simulink model "sim_all"  (R2020a)
settings: Solver=VariableStepAuto  StartTime=0.0  StopTime=2000  RelTol=1e-3
undefined symbols (not defined in the file or in its folder): a1, a2, alpha1, alpha2, cornerA, cornerB, cornerC, cornerD, ctrl_clockwise, ctrl_int_bound_or, ctrl_int_bound_pos, ctrl_k_or, ctrl_k_pos, ctrl_Ki_vel, ctrl_Kp_v_pos, ctrl_Kp_vel, ctrl_TAM, ctrl_Ts, ctrl_va_uncontrolled, ctrl_vel_uncontrolled, D, dead_zone_limit, depth, DiscIntNeverNeededParam, distanceFromWall, initInspectedSide, initPoint, mod_A, mod_Cd_F, mod_Cd_M, mod_eta_init, mod_g, mod_h0, mod_Ixx, mod_Iyy, mod_Izz, mod_Kp_dot, mod_lat0, mod_lon0, mod_m, mod_Mq_dot, mod_ni_init, mod_Nr_dot, mod_p1, mod_p2, mod_p3, mod_p4, mod_p5, mod_p6, mod_R, mod_Rm, mod_t1, mod_t2, mod_t3, mod_t4, mod_t5, mod_t6, mod_W, mod_Xu_dot, mod_Yv_dot ... (+53)
libraries: simulink x8, cstblocks x6, simulink_extras x1
(part 3 of 6)

== system sim_all/Mission_supervisor_v3/Mission_Supervisor/Orientazione Iniziale ==
  Pos_s : Inport
  Or_s : Inport  Port=2
  Or_in : Inport  Port=3
  error_flag : Inport  Port=4
  Action Port : ActionPort  ActionPortLabel=case [ 101 ]:
  Constant{,1..3} (4 alike) : Constant  Value=nan
  MATLAB Function : MATLAB Function  TreatAsAtomicUnit=on  SystemSampleTime=Ts_supervisor
  Mux : Mux  Inputs=6
  delta_current_or_iniz : Outport
  delta_stato_or_iniz : Outport  Port=2
  Outport : Outport  Port=3
  wires:
  MATLAB Function/2(delta_current_or_iniz) -> delta_current_or_iniz/1
  MATLAB Function/1(delta_stato_or_iniz) -> delta_stato_or_iniz/1
  Mux/1 -> Outport/1
  Constant/1 -> Mux/3
  Constant1/1 -> Mux/4
  Constant2/1 -> Mux/5
  Constant3/1 -> Mux/6
  Pos_s/1 -> MATLAB Function/1(Pos_s)
  Or_s/1 -> MATLAB Function/2(Or_s)
  Or_in/1 -> MATLAB Function/3(Or_in)
  MATLAB Function/3(Pos_d) -> Mux/1
  MATLAB Function/4(Or_d) -> Mux/2
  error_flag/1 -> MATLAB Function/4(error_flag)

== system sim_all/Mission_supervisor_v3/Mission_Supervisor/Orientazione in profondità ==
  Pos_s : Inport
  Orp_s : Inport  Port=2
  Punto_iniz_patt : Inport  Port=3
  error_flag : Inport  Port=4
  Action Port : ActionPort  ActionPortLabel=case [ 104 ]:
  Constant{,1..3,6} (5 alike) : Constant  Value=nan
  MATLAB Function : MATLAB Function  TreatAsAtomicUnit=on  SystemSampleTime=Ts_supervisor
  Mux : Mux  Inputs=6
  Mux1 : Mux  Inputs=3
  delta_current_or_prof : Outport
  delta_stato_or_prof : Outport  Port=2
  Outport : Outport  Port=3
  wires:
  MATLAB Function/1(delta_current_or_prof) -> delta_current_or_prof/1
  MATLAB Function/2(delta_stato_or_prof) -> delta_stato_or_prof/1
  MATLAB Function/3(Pos_d) -> Mux/1
  Mux/1 -> Outport/1
  Constant1/1 -> Mux/3
  MATLAB Function/4(Dpp_d) -> Mux/4
  MATLAB Function/5(Orp_d) -> Mux/6
  Constant/1 -> Mux1/1
  Constant2/1 -> Mux1/2
  Constant6/1 -> Mux1/3
  Mux1/1 -> Mux/2
  Constant3/1 -> Mux/5
  Pos_s/1 -> MATLAB Function/1(Pos_s)
  Orp_s/1 -> MATLAB Function/2(Orp_s)
  Punto_iniz_patt/1 -> MATLAB Function/3(punto_iniz_patt)
  error_flag/1 -> MATLAB Function/4(error_flag)

== system sim_all/Mission_supervisor_v3/Mission_Supervisor/Orientazione in superficie ==
  Or_in : Inport
  error_flag : Inport  Port=2
  punto_iniz_patt : Inport  Port=3
  Pos_s : Inport  Port=4
  Or_s : Inport  Port=5
  Action Port : ActionPort  ActionPortLabel=case [ 302 ]:
  Constant{1..2,4..5} (4 alike) : Constant  Value=nan
  MATLAB Function : MATLAB Function  TreatAsAtomicUnit=on  SystemSampleTime=Ts_supervisor
  Mux : Mux  Inputs=6
  delta_current_or_sup : Outport
  delta_stato_or_sup : Outport  Port=2
  Outport : Outport  Port=3
  wires:
  Mux/1 -> Outport/1
  Constant1/1 -> Mux/3
  Constant4/1 -> Mux/5
  Or_in/1 -> MATLAB Function/1(Or_in)
  error_flag/1 -> MATLAB Function/2(error_flag)
  punto_iniz_patt/1 -> MATLAB Function/3(punto_iniz_patt)
  MATLAB Function/1(delta_current_or_sup) -> delta_current_or_sup/1
  MATLAB Function/2(delta_stato_or_sup) -> delta_stato_or_sup/1
  MATLAB Function/4(Or_d) -> Mux/2
  MATLAB Function/3(Pos_d) -> Mux/1
  Constant2/1 -> Mux/4
  Constant5/1 -> Mux/6
  Pos_s/1 -> MATLAB Function/4(Pos_s)
  Or_s/1 -> MATLAB Function/5(Or_s)

== system sim_all/Mission_supervisor_v3/Mission_Supervisor/Pattugliamento ==
  parete : Inport
  contatore : Inport  Port=2
  Pos_s : Inport  Port=3
  Dpp_s : Inport  Port=4
  Dps_s : Inport  Port=5
  Orp_s : Inport  Port=6
  Vel_s : Inport  Port=7
  error_flag : Inport  Port=8
  giro : Inport  Port=9
  Action Port : ActionPort  ActionPortLabel=case [ 201 ]:
  Constant{,1..2,6} (4 alike) : Constant  Value=nan
  MATLAB Function : MATLAB Function  TreatAsAtomicUnit=on  SystemSampleTime=Ts_supervisor
  Mux : Mux  Inputs=6
  Mux1 : Mux  Inputs=3
  delta_current_patt : Outport
  delta_stato_patt : Outport  Port=2
  Outport : Outport  Port=3
  wires:
  MATLAB Function/1(delta_current_patt) -> delta_current_patt/1
  MATLAB Function/2(delta_stato_patt) -> delta_stato_patt/1
  parete/1 -> MATLAB Function/1(parete)
  contatore/1 -> MATLAB Function/2(contatore)
  MATLAB Function/3(Pos_d) -> Mux/1
  Mux/1 -> Outport/1
  Mux1/1 -> Mux/2
  MATLAB Function/4(Vel_d) -> Mux/3
  MATLAB Function/5(Dpp_d) -> Mux/4
  Constant/1 -> Mux1/1
  Constant2/1 -> Mux1/2
  Constant6/1 -> Mux1/3
  Pos_s/1 -> MATLAB Function/3(Pos_s)
  Dpp_s/1 -> MATLAB Function/4(Dpp_s)
  Dps_s/1 -> MATLAB Function/5(Dps_s)
  Vel_s/1 -> MATLAB Function/7(Vel_s)
  Orp_s/1 -> MATLAB Function/6(Orp_s)
  error_flag/1 -> MATLAB Function/8(error_flag)
  giro/1 -> MATLAB Function/9(giro)
  Constant1/1 -> Mux/5
  MATLAB Function/6(Orp_d) -> Mux/6

== system sim_all/Mission_supervisor_v3/Mission_Supervisor/Posizionamento ==
  Pos_s : Inport
  Or_s : Inport  Port=2
  punto iniziale : Inport  Port=3
  Or_in : Inport  Port=4
  error_flag : Inport  Port=5
  Action Port : ActionPort  ActionPortLabel=case [ 102 ]:
  Constant{,1..3} (4 alike) : Constant  Value=nan
  MATLAB Function : MATLAB Function  TreatAsAtomicUnit=on  SystemSampleTime=Ts_supervisor
  Mux : Mux  Inputs=6
  delta_current_posiz : Outport
  delta_stato_posiz : Outport  Port=2
  Outport : Outport  Port=3
  wires:
  MATLAB Function/1(delta_current_posiz) -> delta_current_posiz/1
  MATLAB Function/2(delta_stato_posiz) -> delta_stato_posiz/1
  MATLAB Function/3(Pos_d) -> Mux/1
  MATLAB Function/4(Or_d) -> Mux/2
  Mux/1 -> Outport/1
  Constant/1 -> Mux/3
  Constant1/1 -> Mux/6
  Constant2/1 -> Mux/5
  Pos_s/1 -> MATLAB Function/1(Pos_s)
  punto iniziale/1 -> MATLAB Function/3(punto_iniziale)
  Or_in/1 -> MATLAB Function/4(Or_in)
  Or_s/1 -> MATLAB Function/2(Or_s)
  error_flag/1 -> MATLAB Function/5(error_flag)
  Constant3/1 -> Mux/4

== system sim_all/Mission_supervisor_v3/Mission_Supervisor/Rientro ==
  Pos_s : Inport
  Or_in : Inport  Port=2
  error_flag : Inport  Port=3
  Dps_s : Inport  Port=4
  Dpp_s : Inport  Port=5
  Or_s : Inport  Port=6
  Action Port : ActionPort  ActionPortLabel=case [ 303 ]:
  Constant{1..4} (4 alike) : Constant  Value=nan
  MATLAB Function : MATLAB Function  TreatAsAtomicUnit=on  SystemSampleTime=Ts_supervisor
  Mux : Mux  Inputs=6
  delta_current_rient : Outport
  delta_stato_rient : Outport  Port=2
  Outport : Outport  Port=3
  wires:
  MATLAB Function/1(delta_current_rient) -> delta_current_rient/1
  MATLAB Function/2(delta_stato_rient) -> delta_stato_rient/1
  MATLAB Function/3(Pos_d) -> Mux/1
  Mux/1 -> Outport/1
  Constant1/1 -> Mux/3
  Constant2/1 -> Mux/4
  Constant3/1 -> Mux/5
  Constant4/1 -> Mux/6
  Pos_s/1 -> MATLAB Function/1(Pos_s)
  MATLAB Function/4(Or_d) -> Mux/2
  Or_in/1 -> MATLAB Function/2(Or_in)
  error_flag/1 -> MATLAB Function/3(error_flag)
  Dps_s/1 -> MATLAB Function/4(Dps_s)
  Dpp_s/1 -> MATLAB Function/5(Dpp_s)
  Or_s/1 -> MATLAB Function/6(Or_s)

== system sim_all/Mission_supervisor_v3/Mission_Supervisor/Risalita ==
  delta_SOS : Inport
  Pos_s : Inport  Port=2
  Dpp_s : Inport  Port=3
  Orp_s : Inport  Port=4
  Dps_s : Inport  Port=5
  Dps_fin : Inport  Port=6
  error_flag : Inport  Port=7
  SOS_205 : Inport  Port=8
  Action Port : ActionPort  ActionPortLabel=case [ 301 ]:
  Constant{,1,3,6} (4 alike) : Constant  Value=nan
  MATLAB Function : MATLAB Function  TreatAsAtomicUnit=on  SystemSampleTime=Ts_supervisor
  Mux : Mux  Inputs=6
  Mux1 : Mux  Inputs=3
  delta_current_ris : Outport
  delta_stato_ris : Outport  Port=2
  Outport : Outport  Port=3
  wires:
  MATLAB Function/1(delta_current_ris) -> delta_current_ris/1
  MATLAB Function/2(delta_stato_ris) -> delta_stato_ris/1
  MATLAB Function/3(Pos_d) -> Mux/1
  Mux/1 -> Outport/1
  Mux1/1 -> Mux/2
  Constant1/1 -> Mux/3
  MATLAB Function/4(Dpp_d) -> Mux/4
  Constant/1 -> Mux1/1
  Constant3/1 -> Mux1/2
  Constant6/1 -> Mux1/3
  MATLAB Function/5(Dps_d) -> Mux/5
  Pos_s/1 -> MATLAB Function/2(Pos_s)
  Dpp_s/1 -> MATLAB Function/3(Dpp_s)
  MATLAB Function/6(Orp_d) -> Mux/6
  delta_SOS/1 -> MATLAB Function/1(delta_SOS)
  Orp_s/1 -> MATLAB Function/4(Orp_s)
  Dps_s/1 -> MATLAB Function/5(Dps_s)
  Dps_fin/1 -> MATLAB Function/6(Dps_fin)
  error_flag/1 -> MATLAB Function/7(error_flag)
  SOS_205/1 -> MATLAB Function/8(SOS_205)

== system sim_all/Model/Vehicle Model/P1 ==
  note: n is the rotational speed of the thruster
      | V is the speed component of the water along the thruster axis
      |
      | n is saturated according to data
      | a dead zone is considered according to data
      | the thruster is characterised by 1st order dynamics (tau = 0.2s)
  n1 [rad/s] : Inport
  V1 [m/s] : Inport  Port=2
  Dead Zone : DeadZone  LowerValue=-dead_zone_limit  UpperValue=dead_zone_limit  SaturateOnIntegerOverflow=on
  Propeller1 : MATLAB Function  TreatAsAtomicUnit=on
  Saturation : Saturate  UpperLimit=n_max  LowerLimit=-n_max
  Transfer Fcn : TransferFcn  Denominator=[0.2 1]
  T1 : Outport
  wires:
  V1 [m/s]/1 -> Propeller1/2(V1)
  Saturation/1 -> Propeller1/1(n1)
  Transfer Fcn/1 -> Saturation/1
  Dead Zone/1 -> Transfer Fcn/1
  n1 [rad/s]/1 -> Dead Zone/1
  Propeller1/1(T1) -> T1/1

== system sim_all/Model/Vehicle Model/P2 ==
  note: n is the rotational speed of the thruster
      | V is the speed component of the water along the thruster axis
      |
      | n is saturated according to data
      | a dead zone is considered according to data
      | the thruster is characterised by 1st order dynamics (tau = 0.2s)
  n2 [rad/s] : Inport
  V2 [m/s] : Inport  Port=2
  Dead Zone : DeadZone  LowerValue=-dead_zone_limit  UpperValue=dead_zone_limit  SaturateOnIntegerOverflow=on
  Propeller2 : MATLAB Function  TreatAsAtomicUnit=on
  Saturation : Saturate  UpperLimit=n_max  LowerLimit=-n_max
  Transfer Fcn : TransferFcn  Denominator=[0.2 1]
  T2 : Outport
  wires:
  V2 [m/s]/1 -> Propeller2/2(V2)
  Saturation/1 -> Propeller2/1(n2)
  Transfer Fcn/1 -> Saturation/1
  Dead Zone/1 -> Transfer Fcn/1
  n2 [rad/s]/1 -> Dead Zone/1
  Propeller2/1(T2) -> T2/1

== system sim_all/Model/Vehicle Model/P3 ==
  note: n is the rotational speed of the thruster
      | V is the speed component of the water along the thruster axis
      |
      | n is saturated according to data
      | a dead zone is considered according to data
      | the thruster is characterised by 1st order dynamics (tau = 0.2s)
  n3 [rad/s] : Inport
  V3 [m/s] : Inport  Port=2
  Dead Zone : DeadZone  LowerValue=-dead_zone_limit  UpperValue=dead_zone_limit  SaturateOnIntegerOverflow=on
  Propeller3 : MATLAB Function  TreatAsAtomicUnit=on
  Saturation : Saturate  UpperLimit=n_max  LowerLimit=-n_max
  Transfer Fcn : TransferFcn  Denominator=[0.2 1]
  T3 : Outport
  wires:
  V3 [m/s]/1 -> Propeller3/2(V3)
  Saturation/1 -> Propeller3/1(n3)
  Transfer Fcn/1 -> Saturation/1
  Dead Zone/1 -> Transfer Fcn/1
  n3 [rad/s]/1 -> Dead Zone/1
  Propeller3/1(T3) -> T3/1

== system sim_all/Model/Vehicle Model/P4 ==
  note: n is the rotational speed of the thruster
      | V is the speed component of the water along the thruster axis
      |
      | n is saturated according to data
      | a dead zone is considered according to data
      | the thruster is characterised by 1st order dynamics (tau = 0.2s)
  n4 [rad/s] : Inport
  V4 [m/s] : Inport  Port=2
  Dead Zone : DeadZone  LowerValue=-dead_zone_limit  UpperValue=dead_zone_limit  SaturateOnIntegerOverflow=on
  Propeller4 : MATLAB Function  TreatAsAtomicUnit=on
  Saturation : Saturate  UpperLimit=n_max  LowerLimit=-n_max
  Transfer Fcn : TransferFcn  Denominator=[0.2 1]
  T4 : Outport
  wires:
  V4 [m/s]/1 -> Propeller4/2(V4)
  Saturation/1 -> Propeller4/1(n4)
  Transfer Fcn/1 -> Saturation/1
  Dead Zone/1 -> Transfer Fcn/1
  n4 [rad/s]/1 -> Dead Zone/1
  Propeller4/1(T4) -> T4/1

== system sim_all/Model/Vehicle Model/P5 ==
  note: n is the rotational speed of the thruster
      | V is the speed component of the water along the thruster axis
      |
      | n is saturated according to data
      | a dead zone is considered according to data
      | the thruster is characterised by 1st order dynamics (tau = 0.2s)
  n5 [rad/s] : Inport
  V5 [m/s] : Inport  Port=2
  Dead Zone : DeadZone  LowerValue=-dead_zone_limit  UpperValue=dead_zone_limit  SaturateOnIntegerOverflow=on
  Propeller5 : MATLAB Function  TreatAsAtomicUnit=on
  Saturation : Saturate  UpperLimit=n_max  LowerLimit=-n_max
  Transfer Fcn : TransferFcn  Denominator=[0.2 1]
  T5 : Outport
  wires:
  V5 [m/s]/1 -> Propeller5/2(V5)
  Saturation/1 -> Propeller5/1(n5)
  Transfer Fcn/1 -> Saturation/1
  Dead Zone/1 -> Transfer Fcn/1
  n5 [rad/s]/1 -> Dead Zone/1
  Propeller5/1(T5) -> T5/1

== system sim_all/Model/Vehicle Model/P6 ==
  note: n is the rotational speed of the thruster
      | V is the speed component of the water along the thruster axis
      |
      | n is saturated according to data
      | a dead zone is considered according to data
      | the thruster is characterised by 1st order dynamics (tau = 0.2s)
  n6 [rad/s] : Inport
  V6 [m/s] : Inport  Port=2
  Dead Zone : DeadZone  LowerValue=-dead_zone_limit  UpperValue=dead_zone_limit  SaturateOnIntegerOverflow=on
  Propeller6 : MATLAB Function  TreatAsAtomicUnit=on
  Saturation : Saturate  UpperLimit=n_max  LowerLimit=-n_max
  Transfer Fcn : TransferFcn  Denominator=[0.2 1]
  T6 : Outport
  wires:
  V6 [m/s]/1 -> Propeller6/2(V6)
  Saturation/1 -> Propeller6/1(n6)
  Transfer Fcn/1 -> Saturation/1
  Dead Zone/1 -> Transfer Fcn/1
  n6 [rad/s]/1 -> Dead Zone/1
  Propeller6/1(T6) -> T6/1

== system sim_all/Navigation/Extended Kalman Filter/AHRS__check ==
  AHRS_new : Inport
  MATLAB Function4 : MATLAB Function  TreatAsAtomicUnit=on
  Memory4 : Memory
  flag_AHRS : Outport
  AHRS_now : Outport  Port=2
  wires:
  AHRS_new/1 -> MATLAB Function4/1(AHRS_new)
  Memory4/1 -> MATLAB Function4/2(AHRS_old)
  MATLAB Function4/1(flag_AHRS) -> flag_AHRS/1
  MATLAB Function4/2(AHRS_now) -> Memory4/1, AHRS_now/1

== system sim_all/Navigation/Extended Kalman Filter/CORREZIONE ==
  x_k|k-1 : Inport
  P_k|k-1 : Inport  Port=2
  e : Inport  Port=3
  H : Inport  Port=4
  R : Inport  Port=5
  nav_flag_init : Inport  Port=6
  MATLAB Function : MATLAB Function  TreatAsAtomicUnit=on  SystemSampleTime=nav_DT
  x_k|k : Outport
  P_k|k : Outport  Port=2
  wires:
  x_k|k-1/1 -> MATLAB Function/1(x_k_k_1)
  P_k|k-1/1 -> MATLAB Function/2(P_k_k_1)
  e/1 -> MATLAB Function/3(e)
  H/1 -> MATLAB Function/4(H)
  MATLAB Function/1(x_k) -> x_k|k/1
  MATLAB Function/2(P_k) -> P_k|k/1
  nav_flag_init/1 -> MATLAB Function/6(nav_flag_init)
  R/1 -> MATLAB Function/5(R_k)

== system sim_all/Navigation/Extended Kalman Filter/DVL_check ==
  DVL_new : Inport
  MATLAB Function4 : MATLAB Function  TreatAsAtomicUnit=on
  Memory4 : Memory
  flag_DVL : Outport
  DVL_now : Outport  Port=2
  wires:
  DVL_new/1 -> MATLAB Function4/1(DVL_new)
  Memory4/1 -> MATLAB Function4/2(DVL_old)
  MATLAB Function4/1(flag_DVL) -> flag_DVL/1
  MATLAB Function4/2(DVL_now) -> Memory4/1, DVL_now/1

== system sim_all/Navigation/Extended Kalman Filter/MISURA VIRTUALE ==
  x_k|k-1 : Inport
  flag_vect : Inport  Port=2
  mis_vect : Inport  Port=3
  J : Inport  Port=4
  MATLAB Function : MATLAB Function  TreatAsAtomicUnit=on  SystemSampleTime=nav_DT
  e : Outport
  H : Outport  Port=2
  wires:
  x_k|k-1/1 -> MATLAB Function/1(x_k_k_1)
  mis_vect/1 -> MATLAB Function/3(mis_vect)
  flag_vect/1 -> MATLAB Function/2(flag_vect)
  MATLAB Function/1(e) -> e/1
  MATLAB Function/2(H) -> H/1
  J/1 -> MATLAB Function/4(J)

== system sim_all/Navigation/Extended Kalman Filter/PREDIZIONE ==
  x0 : Inport
  P0 : Inport  Port=2
  x_k-1|k-1 : Inport  Port=3
  u_k-1 : Inport  Port=4
  P_k-1|k-1 : Inport  Port=5
  J : Inport  Port=6
  L : Inport  Port=7
  Q_k-1 : Inport  Port=8
  nav_flag_init : Inport  Port=9
  Passo di Predizione : MATLAB Function  TreatAsAtomicUnit=on  SystemSampleTime=nav_DT
  x_k|k-1 : Outport
  P_k|k-1 : Outport  Port=2
  flag_init : Outport  Port=3
  wires:
  Passo di Predizione/1(x_k) -> x_k|k-1/1
  Passo di Predizione/2(P_k) -> P_k|k-1/1
  u_k-1/1 -> Passo di Predizione/4(u_k_1)
  x_k-1|k-1/1 -> Passo di Predizione/3(x_k_1)
  P_k-1|k-1/1 -> Passo di Predizione/5(P_k_1)
  J/1 -> Passo di Predizione/6(J)
  Q_k-1/1 -> Passo di Predizione/8(Q_k_1)
  P0/1 -> Passo di Predizione/2(P0)
  x0/1 -> Passo di Predizione/1(x0)
  L/1 -> Passo di Predizione/7(L)
  nav_flag_init/1 -> Passo di Predizione/9("nav_flag_init ")
  Passo di Predizione/3(nav_flag_init) -> flag_init/1

== system sim_all/Navigation/Extended Kalman Filter/Q_error ==
  flag_AHRS : Inport
  flag_DVL : Inport  Port=2
  Q : Inport  Port=3
  MATLAB Function4 : MATLAB Function  TreatAsAtomicUnit=on
  Memory : Memory
  Q_k : Outport
  wires:
  MATLAB Function4/1(Q_k) -> Q_k/1, Memory/1
  flag_AHRS/1 -> MATLAB Function4/3(flag_AHRS)
  flag_DVL/1 -> MATLAB Function4/4(flag_DVL)
  Memory/1 -> MATLAB Function4/2(Q_k_1)
  Q/1 -> MATLAB Function4/1(Q)

== system sim_all/Sensors/BLOCCO GYRO1/Subsystem ==
  t : Inport  SampleTime=sens_Sample_time_GYRO
  GEOD to NED : MATLAB Function  TreatAsAtomicUnit=on
  Bias_G : Outport
  wires:
  t/1 -> GEOD to NED/1(t)
  GEOD to NED/1(Bias_G) -> Bias_G/1

== matlab function sim_all/Navigation/Extended Kalman Filter/AHRS__check/MATLAB Function4 ==
  data: flag_AHRS output; AHRS_new input; AHRS_now output; AHRS_old input
%gestione di misura errata di AHRS
function [flag_AHRS, AHRS_now] = fcn(AHRS_new, AHRS_old)

    if isnan(AHRS_new(1,1)) || isnan(AHRS_new(2,1)) || isnan(AHRS_new(3,1))
        AHRS_now = AHRS_old;
        flag_AHRS = 1;
        disp('Misura AHRS non valida')
    else
        AHRS_now = AHRS_new;
        flag_AHRS = 0;
    end  
end

== matlab function sim_all/Navigation/Extended Kalman Filter/CORREZIONE/MATLAB Function ==
  data: x_k_k_1 input; x_k output; P_k_k_1 input; e input size=6 1; H input size=6 3; R_k input size=6 6; P_k output; nav_flag_init input
%%Passo di Correzione

function [x_k, P_k] = correction(x_k_k_1,P_k_k_1, e, H, R_k,nav_flag_init)
    
     x_k = zeros(3,1);
     P_k = zeros(3,3);
     
     
    if nav_flag_init ~= 0
        %matrice ottenuta da derivata di funzione h (6x1) per i rumori sei vari
        %sensori, che sono 6. (ha dimensione 6x6)
        %andrebbero anche considerati i rumori legati all'AHRS che al momento
        %sono trascurati
        %M = eye(6,6);              %M è l'dientità
        S_k = H*P_k_k_1*H'+ R_k;
        K_k = P_k_k_1*H'*(inv(S_k));

        P_k = (eye(3)-(K_k*H))*P_k_k_1;
        x_k = x_k_k_1 + K_k * e;
    end

end

== matlab function sim_all/Navigation/Extended Kalman Filter/Creazione vettore delle misure ==
  data: flag_vect output; GPS input; mis_vect output; depth input; s_pr input; s_dx input; s_sx input; mis_vect_prec input; J input; pos input; nav_plane_AB parameter; nav_plane_BC parameter; nav_plane_CD parameter; nav_plane_DA parameter; nav_A parameter; nav_B parameter; nav_C parameter; nav_D parameter; distanceFromWall parameter; flag_DVL input; flag_AHRS input
%%
% Questa funzione impila le informazioni derivanti dai vari sensori in un
% unico vettore mis_vect 7x1.                                 
% Ci sarà un corrispondente vettore flag_vect 7x1 di flag che sarà pari a:

% flag(i) = 0  se la misura è uguale a quella arrivata nell'istante
% predecente, in tal caso la correzione non verrà effettuata
% flag(i) = 1 se la misura è stata aggiornata rispetto a quella precendente
 
% NB il controllo sulla validità dei dati del GPS è valutata nel blocco
% sucessivo

function [flag_vect,mis_vect] = misure_vector(GPS,depth,s_pr,s_dx,s_sx, mis_vect_prec,...
          J, pos, nav_plane_AB, nav_plane_BC, nav_plane_CD, nav_plane_DA, nav_A, nav_B, nav_C, nav_D, distanceFromWall, ...
          flag_DVL, flag_AHRS)
    
    mis_vect = zeros(7,1);
    flag_vect = zeros(7,1);
	mis_vect = [GPS(1) GPS(2) GPS(3) depth s_pr s_dx s_sx]';
    
    for i=[1:7]
        if mis_vect(i) ~= mis_vect_prec(i)
            flag_vect(i) = 1;
        end
    end
    
    %si valuta se la misura del profondimetro è valida
    if isnan(depth)  
        flag_vect(4) = 0;
    end
     
    %si controlla che sia disponibile il dato dai sonar
    if isnan(s_pr)
        flag_vect(5) = 0;
    end
    if isnan(s_dx)
        flag_vect(6) = 0;
    end
    if isnan(s_sx)
        flag_vect(7) = 0;
    end
    
    %se i dati dei sonar qui sono utilizzabili, è necessario assicurarci che il 
    %loro raggio non punti verso uno spigolo, in quel caso potrebbe
    %causare una correzione errata
    if flag_vect(5) == 1               %se i dati del sonar di prua sono nuovi
            versore_son_NED = J*[1 0 0]';          %versore terna NED sonar prua
            flag_vect(5) = inter(pos, versore_son_NED ,nav_plane_AB,nav_plane_BC,nav_plane_CD,nav_plane_DA, nav_A, nav_B, nav_C, nav_D);       
    end

        if flag_vect(6) == 1               %se i dati del sonar destro sono nuovi
                versore_son_NED = J*[0 1 0]';          %versore terna NED sonar dx
                flag_vect(6) = inter(pos, versore_son_NED ,nav_plane_AB,nav_plane_BC,nav_plane_CD,nav_plane_DA, nav_A, nav_B, nav_C, nav_D);       
        end
        if flag_vect(7) == 1               %se i dati del sonar sinistro sono nuovi
                versore_son_NED = J*[0 -1 0]';          %versore terna NED sonar sx
                flag_vect(7) = inter(pos, versore_son_NED ,nav_plane_AB,nav_plane_BC,nav_plane_CD,nav_plane_DA, nav_A, nav_B, nav_C, nav_D);
        end 
%         la terza componente di flag_vect non sarà utilizzata. per assicurarci
%         che i dati del GPS siano validi ci rifaremo sempre su mis_vect


    if flag_DVL == 0 && flag_AHRS == 0  %i sonar vengono usati sempre nella correzione se un sensore tra DLV
                                        %o AHRS non funziona momentaneamente 
        
        soglia_distanza=distanceFromWall*3;
        soglia_variazione=0.8;
        if  mis_vect(5) > soglia_distanza || abs(mis_vect(5)- mis_vect_prec(5)) > soglia_variazione
            flag_vect(5) = 0;
        end
        if  mis_vect(6) > soglia_distanza || abs(mis_vect(6)- mis_vect_prec(6)) > soglia_variazione
            flag_vect(6) = 0;
        end
        if  mis_vect(7) > soglia_distanza || abs(mis_vect(7)- mis_vect_prec(7)) > soglia_variazione
            flag_vect(7) = 0;
        end
    end
end




function [flag] = inter(pos, versore_son_NED,nav_plane_AB,nav_plane_BC,nav_plane_CD,nav_plane_DA, nav_A, nav_B, nav_C, nav_D)
    
    %calcolo della distanza dalla posizione ai piani delle pareti seguendo
    %la direzione data dal versore del sonar

    t_AB = -(pos(1)+nav_plane_AB(2)*pos(2)+nav_plane_AB(4))/(nav_plane_AB(2)*versore_son_NED(2)+versore_son_NED(1));
    t_BC = -(pos(1)+nav_plane_BC(2)*pos(2)+nav_plane_BC(4))/(nav_plane_BC(2)*versore_son_NED(2)+versore_son_NED(1));
    t_CD = -(pos(1)+nav_plane_CD(2)*pos(2)+nav_plane_CD(4))/(nav_plane_CD(2)*versore_son_NED(2)+versore_son_NED(1));
    t_DA = -(pos(1)+nav_plane_DA(2)*pos(2)+nav_plane_DA(4))/(nav_plane_DA(2)*versore_son_NED(2)+versore_son_NED(1));
    
    if t_AB < 0
        t_AB = inf;
    end
    if t_BC < 0
        t_BC = inf;
    end
    if t_CD < 0
        t_CD = inf;
    end
    if t_DA < 0
        t_DA = inf;
    end
           
    [dist, index] = min([t_AB t_BC t_CD t_DA]);
    dist = dist - 0.267;       %va tolto il raggio del veicolo rispetto al centro di massa
    
    int=zeros(1,3);
    %calcolo l'intersezione
    int(1) = pos(1) + versore_son_NED(1)*dist;
    int(2) = pos(2) + versore_son_NED(2)*dist;
    int(3) = 0;
    
    soglia_spigolo = 5;          %distanza massima dallo spigolo entro la quale 
                       %la misura del sonar non è buona
    flag=1;
    switch index
        case 1      
            if norm(int-nav_A) < soglia_spigolo || norm(int-nav_B) < soglia_spigolo
                flag=0;
            end
        case 2
            if norm(int-nav_B) < soglia_spigolo || norm(int-nav_C) < soglia_spigolo
                flag=0;
            end
        case 3
            if norm(int-nav_C) < soglia_spigolo || norm(int-nav_D) < soglia_spigolo
                flag=0;
            end
        case 4
            if norm(int-nav_D) < soglia_spigolo || norm(int-nav_A) < soglia_spigolo
                flag=0;
            end
        otherwise
            disp('errore nella intersezione del piano')
    end
end

== matlab function sim_all/Mission_supervisor_v3/Mission_Supervisor/Orientazione Iniziale/MATLAB Function ==
  data: delta_stato_or_iniz output; delta_current_or_iniz output; Pos_d output size=3; Pos_s input size=3; Or_s input size=3; Or_in input; initPoint parameter size=3; Or_d output size=3; error_flag input; soglia_or parameter; soglia_SOS_pos parameter; SOS parameter; soglia_SOS_or parameter
function [delta_stato_or_iniz, delta_current_or_iniz, Pos_d, Or_d] = Orientazione_iniziale(Pos_s, Or_s, Or_in, initPoint, error_flag, soglia_or, soglia_SOS_pos, SOS, soglia_SOS_or)

    disp("Orientazione iniziale");
    
    %% Unità di misura 
    
    % Pos_d, Pos_s, initPoint, soglia_SOS_pos                                [deg, deg, m]
    % Or_d, Or_s, Or_in, soglia_or, soglia_SOS_or                            [rad, rad, rad]
    
    %% Inizializzazione variabili
    
    % Mantenimento dello stato_interno al valore
    % desiderato durante la permanenza del sistema nello stato corrente.
    delta_stato_or_iniz = 0;
    
    % Variabile utilizzata per segnalare il momento in cui
    % effettuare la transizione di stato. 
    pronti = false;
    
    %% Preparazione dei riferimenti da fornire ai blocchi successivi
                
    % Posizione da mantenere
    Pos_d = initPoint; 
   
    % Orientazione desiderata per raggiungere
    % il punto di inizio pattugliamento
    Or_d = Or_in;
    
    % Quando i riferimenti sono correttamente settati
    % il passaggio di stato viene comunicato agli altri moduli
    delta_current_or_iniz = 101 - 100;
    
    
    %% Verifiche
    
    % Si verifica il mantenimento della posizione 
    % e la ricezione della stima di orientazione
    if (abs(Pos_s(1) - Pos_d(1)) > soglia_SOS_pos(1) || ...
        abs(Pos_s(2) - Pos_d(2)) > soglia_SOS_pos(2) || ...
        abs(Pos_s(3) - Pos_d(3)) > soglia_SOS_pos(3) || ...
        isnan(Or_s(1)) || isnan(Or_s(2)) || isnan(Or_s(3)) || ...
        abs(Or_s(1) - Or_d(1)) > soglia_SOS_or(1) || ...
        abs(Or_s(2) - Or_d(2)) > soglia_SOS_or(2))
    
        SOS = 1;
        disp("EMERGENZA:");
        
        if (abs(Pos_s(1) - Pos_d(1)) > soglia_SOS_pos(1))
            disp("Rilevato errore sulla posizione X");
        end
        if (abs(Pos_s(2) - Pos_d(2)) > soglia_SOS_pos(2))
            disp("Rilevato errore sulla posizione Y");
        end
        if (abs(Pos_s(3) - Pos_d(3)) > soglia_SOS_pos(3))
            disp("Rilevato errore sulla profondita Z");
        end
        if (isnan(Or_s(1)))
            disp("Mancata ricezione della prima componente di orientazione");
        end
        if (isnan(Or_s(2)))
            disp("Mancata ricezione della seconda componente di orientazione");
        end
        if (isnan(Or_s(3)))
            disp("Mancata ricezione della terza componente di orientazione");
        end
        if (abs(Or_s(1) - Or_d(1)) > soglia_SOS_or(1))
            disp("Rilevato errore sulla rotazione di roll");
        end
        if (abs(Or_s(2) - Or_d(2)) > soglia_SOS_or(2))
            disp("Rilevato errore sulla rotazione di pitch");
        end
    end

    if error_flag == 1
        disp("EMERGENZA: errore segnalato dagli altri sottosistemi");
        SOS = 1;
    end
    
    % Si verifica di aver raggiunto l'orientazione desiderata
    if (SOS == 0 && ...
        (abs(Or_s(3) - Or_d(3)) < soglia_or(3)))
    
        pronti = true;
        
    end
       
    %% Decisione dello stato successivo
    
    if pronti == true
        
        delta_stato_or_iniz = 102 - 101; % Transizione eseguita correttamente
    end
        
    if SOS == 1
            
            delta_stato_or_iniz = 304 - 101; % Transizione nello stato di emergenza
    end
    % Si rimane nello stato corrente

end

== matlab function sim_all/Navigation/Extended Kalman Filter/DVL_check/MATLAB Function4 ==
  data: flag_DVL output; DVL_new input; DVL_now output; DVL_old input
%gestione di misura errata del DVL
function [flag_DVL, DVL_now] = fcn(DVL_new, DVL_old)

    if isnan(DVL_new(1,1)) || isnan(DVL_new(2,1)) || isnan(DVL_new(3,1))
        DVL_now = DVL_old;
        flag_DVL = 1;
        disp('Misura DVL non valida')
    else
        DVL_now = DVL_new;
        flag_DVL = 0;
    end  
end

== matlab function sim_all/Navigation/Extended Kalman Filter/MATLAB Function ==
  data: GPS input; x0 output; depth input; P0 output; flag input; flag output
%blocco di inizializzazione del Filtro

function [x0, P0, flag] = EKF_init(GPS, depth, flag)
    
    x0 = zeros(3,1);
    P0 = zeros(3,3);
    
    % il valore di nav_flag_init è all'inizio della simulazione pari a 0
    % appena c'è il primo dato disponibile del GPS (insieme al profondimetro)
    % si assume quella come punto di inizializzazione del filtro.

    if flag == 0
        if GPS(3)==1
            x0 = [GPS(1), GPS(2), depth]';
            P0 = diag([3 3 (0.2)^2]);       %sono le varianze del GPS e del profondimetro (come nella R)
            flag = 1;                   %se vale 1 bisogna assegnare i primi valori a x_k_1 e P_k_1
        end
               
    end

end

== matlab function sim_all/Navigation/Extended Kalman Filter/MATLAB Function1 ==
  data: orient input; J output
%calcolo matrice J
function J = calcolo_jacobiano(orient)

    Roll  = orient(1);
    Pitch = orient(2);
    Yaw   = orient(3);

    R_x = [ 1               0              0;
            0           cos(Roll)     sin(Roll);
            0           -sin(Roll)    cos(Roll)];

    R_y = [cos(Pitch)       0   -sin(Pitch);
              0             1         0;
           sin(Pitch)       0   cos(Pitch)];

    R_z = [cos(Yaw)     sin(Yaw)      0;
          -sin(Yaw)     cos(Yaw)      0;
              0            0          1];

    J = (R_z'*R_y')*R_x';
end

== matlab function sim_all/Navigation/Extended Kalman Filter/MATLAB Function2 ==
  data: u_k_1 input; orient input; L output
%calcolo matrice L
function L = calcolo_L(u_k_1,orient)

    L =  [   u_k_1(2)*((sin(orient(1))*sin(orient(3)))/10 + (cos(orient(1))*cos(orient(3))*sin(orient(2)))/10) + u_k_1(3)*((cos(orient(1))*sin(orient(3)))/10 - (cos(orient(3))*sin(orient(1))*sin(orient(2)))/10), (u_k_1(3)*cos(orient(1))*cos(orient(3))*cos(orient(2)))/10 - (u_k_1(1)*cos(orient(3))*sin(orient(2)))/10 + (u_k_1(2)*cos(orient(3))*cos(orient(2))*sin(orient(1)))/10, u_k_1(3)*((cos(orient(3))*sin(orient(1)))/10 - (cos(orient(1))*sin(orient(3))*sin(orient(2)))/10) - u_k_1(2)*((cos(orient(1))*cos(orient(3)))/10 + (sin(orient(1))*sin(orient(3))*sin(orient(2)))/10) - (u_k_1(1)*cos(orient(2))*sin(orient(3)))/10, (cos(orient(3))*cos(orient(2)))/10, (cos(orient(3))*sin(orient(1))*sin(orient(2)))/10 - (cos(orient(1))*sin(orient(3)))/10, (sin(orient(1))*sin(orient(3)))/10 + (cos(orient(1))*cos(orient(3))*sin(orient(2)))/10;...
           - u_k_1(2)*((cos(orient(3))*sin(orient(1)))/10 - (cos(orient(1))*sin(orient(3))*sin(orient(2)))/10) - u_k_1(3)*((cos(orient(1))*cos(orient(3)))/10 + (sin(orient(1))*sin(orient(3))*sin(orient(2)))/10), (u_k_1(3)*cos(orient(1))*cos(orient(2))*sin(orient(3)))/10 - (u_k_1(1)*sin(orient(3))*sin(orient(2)))/10 + (u_k_1(2)*cos(orient(2))*sin(orient(1))*sin(orient(3)))/10, u_k_1(3)*((sin(orient(1))*sin(orient(3)))/10 + (cos(orient(1))*cos(orient(3))*sin(orient(2)))/10) - u_k_1(2)*((cos(orient(1))*sin(orient(3)))/10 - (cos(orient(3))*sin(orient(1))*sin(orient(2)))/10) + (u_k_1(1)*cos(orient(3))*cos(orient(2)))/10, (cos(orient(2))*sin(orient(3)))/10, (cos(orient(1))*cos(orient(3)))/10 + (sin(orient(1))*sin(orient(3))*sin(orient(2)))/10, (cos(orient(1))*sin(orient(3))*sin(orient(2)))/10 - (cos(orient(3))*sin(orient(1)))/10;...
                                                                                                             (u_k_1(2)*cos(orient(1))*cos(orient(2)))/10 - (u_k_1(3)*cos(orient(2))*sin(orient(1)))/10,                                      - (u_k_1(1)*cos(orient(2)))/10 - (u_k_1(3)*cos(orient(1))*sin(orient(2)))/10 - (u_k_1(2)*sin(orient(1))*sin(orient(2)))/10,                                                                                                                                                                                                                              0,               -sin(orient(2))/10,                                               (cos(orient(2))*sin(orient(1)))/10,                                               (cos(orient(1))*cos(orient(2)))/10]; 
end

== matlab function sim_all/Navigation/Extended Kalman Filter/MATLAB Function3 ==
  data: flag_vect input; mis_vect input; R_ input size=6 6; R_k output size=6 6
%calcolo matrice R
function R_k = R_cutter(flag_vect, mis_vect,R_)
%valutazione misure GPS
    R=R_;   
    i=0;
    if mis_vect(3) == 0                    %se i dati del GPS non sono validi
        R(1,:) = [];
        R(:,1) = [];
        i=i+1;
        R(2-i,:) = [];
        R(:,2-i) = [];
        i=i+1;
        if flag_vect(4) == 0               %se i dati del profondimetro non sono nuovi
            R(3-i,:) = [];
            R(:,3-i) = [];
            i=i+1;
        end
        if flag_vect(5) == 0               %se i dati del sonar di prua non sono nuovi
            R(4-i,:) = [];
             R(:,4-i) = [];
            i=i+1;
        end
        if flag_vect(6) == 0               %se i dati del sonar sinistro non sono nuovi
            R(5-i,:) = [];
             R(:,5-i) = [];
            i=i+1;
        end
        if flag_vect(7) == 0               %se i dati del sonar destro non sono nuovi
            R(6-i,:) = [];
             R(:,6-i) = [];
        end
    % da qui invece abbiamo il GPS valido
    else
        if flag_vect(1)==0 || flag_vect(2)==0  %se i dati del GPS non sono nuovi
            R(1-i,:) = [];
            R(:,1-i) = [];
            i=i+1;
            R(2-i,:) = [];
            R(:,2-i) = [];
            i=i+1;
        end
       
        if flag_vect(4) == 0               %se i dati del profondimetro non sono nuovi
            R(3-i,:) = [];
            R(:,3-i) = [];
            i=i+1;
        end
       
        R(4-i,:) = []; %annulliamo le misure dei sonar
        R(:,4-i) = [];         
        i=i+1;
        R(5-i,:) = [];
        R(:,5-i) = [];
        i=i+1;
        R(6-i,:) = [];
        R(:,6-i) = [];
       
    end
    R_k=R;
end

== matlab function sim_all/Navigation/Extended Kalman Filter/MISURA VIRTUALE/MATLAB Function ==
  data: x_k_k_1 input; flag_vect input; mis_vect input; e output size=6 1; H output size=6 3; J input; nav_plane_AB parameter; nav_plane_BC parameter; nav_plane_CD parameter; nav_plane_DA parameter
%calcolo  misure virtuali
function [e, H] = virtual(x_k_k_1, flag_vect, mis_vect, J, nav_plane_AB, nav_plane_BC, nav_plane_CD, nav_plane_DA)

    e = zeros(6,1);
    h = zeros(6,1);
    z = zeros(6,1);
    H = zeros(6,3);
    
    
    %valutazione misure GPS
    if mis_vect(3)==1                                   %se i dati del GPS sono validi
        if flag_vect(1) == 1 && flag_vect(2) == 1       %se i dati del GPS sono nuovi
            
            z = z + [mis_vect(1) mis_vect(2) 0 0 0 0]';
            h = h + [x_k_k_1(1)   x_k_k_1(2) 0 0 0 0]';
        
            H(1,:)= [1 0 0];
            H(2,:)= [0 1 0];
        end
    end
    
    %valutazione misure depth
    if flag_vect(4) == 1                                 %se i dati del profondimetro sono nuovi
            
        z = z + [0 0 mis_vect(4) 0 0 0]'; 
        h = h + [0 0  x_k_k_1(3) 0 0 0]';

        H(3,:)= [0 0 1];
    end
    
    %valutiamo ora le misure virtuali solo se quelle del GPS non sono
    %valide
    if mis_vect(3)==0                      %se i dati del GPS non sono validi
        
        if flag_vect(5) == 1               %se i dati del sonar di prua sono nuovi
                
                versore_son_NED = J*[1 0 0]';          %versore terna NED sonar prua
                
                [distanza, plane] = inter(x_k_k_1, versore_son_NED ,nav_plane_AB,nav_plane_BC,nav_plane_CD,nav_plane_DA);
                z = z + [0 0 0 mis_vect(5) 0 0]'; 
                h = h + [0 0 0 distanza    0 0]';
                
                H_new=zeros(1,3);
                [H_new(1), H_new(2), H_new(3)] = calc_H_vect(x_k_k_1, versore_son_NED,plane);
                H(4,:) = H_new;                
        end
    
        if flag_vect(6) == 1               %se i dati del sonar destro sono nuovi
                
                versore_son_NED = J*[0 1 0]';          %versore terna NED sonar dx
                
                [distanza, plane] = inter(x_k_k_1, versore_son_NED ,nav_plane_AB,nav_plane_BC,nav_plane_CD,nav_plane_DA);
                z = z + [0 0 0 0 mis_vect(6) 0]'; 
                h = h + [0 0 0 0 distanza    0]';
                
                H_new=zeros(1,3);
                [H_new(1), H_new(2), H_new(3)] = calc_H_vect(x_k_k_1, versore_son_NED,plane);
                H(5,:) = H_new;
        end
    
        if flag_vect(7) == 1               %se i dati del sonar sinistro sono nuovi
                 
                versore_son_NED = J*[0 -1 0]';          %versore terna NED sonar sx
                
                [distanza, plane] = inter(x_k_k_1, versore_son_NED ,nav_plane_AB,nav_plane_BC,nav_plane_CD,nav_plane_DA);
                z = z + [0 0 0 0 0 mis_vect(7)]'; 
                h = h + [0 0 0 0 0 distanza   ]'; 
                
                H_new=zeros(1,3);
                [H_new(1), H_new(2), H_new(3)] = calc_H_vect(x_k_k_1, versore_son_NED,plane);
                H(6,:) = H_new;
        end
    end
    
    e = z - h;
    
    %%si riducono le dimensioni della matrice H e del vettore e
    
    i=0;
    if mis_vect(3) == 0                    %se i dati del GPS non sono validi
        H(1-i,:) = [];
        e(1-i) = [];
        i=i+1;
        H(2-i,:) = [];
        e(2-i) = [];
        i=i+1;
        if flag_vect(4) == 0               %se i dati del profondimetro non sono nuovi
            H(3-i,:) = [];
            e(3-i) = [];
            i=i+1;
        end
        if flag_vect(5) == 0               %se i dati del sonar di prua non sono nuovi
            H(4-i,:) = [];
            e(4-i) = [];
            i=i+1;
        end
        if flag_vect(6) == 0               %se i dati del sonar sinistro non sono nuovi
            H(5-i,:) = [];
            e(5-i) = [];
            i=i+1;
        end
        if flag_vect(7) == 0               %se i dati del sonar destro non sono nuovi
            H(6-i,:) = [];
            e(6-i) = [];
        end
    % da qui invece si ha il GPS valido
    else
        if flag_vect(1)==0 || flag_vect(2)==0  %se i dati del GPS non sono nuovi
            H(1-i,:) = [];
            e(1-i) = [];
            i=i+1;
            H(2-i,:) = [];
            e(2-i) = [];
            i=i+1;
        end
        
        if flag_vect(4) == 0               %se i dati del profondimetro non sono nuovi
            H(3-i,:) = [];
            e(3-i) = [];
            i=i+1;
        end
        
        H(4-i,:) = [];                      %annulliamo le misure dei sonar
        e(4-i) = [];
        i=i+1;
        H(5-i,:) = [];
        e(5-i) = [];
        i=i+1;
        H(6-i,:) = [];        
        e(6-i) = [];    
    end
    i=0;
end



%%
%%%%%%%%%%%%%%%%%%%%%%%%%%%%%%%%%%%%%%%%%%%%%%%%%%%%%%%%%%%%%%%%%%%%%%%%%%%%%%%%%%%%%%%%

function [dist, plane] = inter(pos, versore_son_NED,nav_plane_AB,nav_plane_BC,nav_plane_CD,nav_plane_DA)
    
    %calcolo della distanza dalla posizione ai piani delle pareti seguendo
    %la direzione data dal versore del sonar

    t_AB = -(pos(1)+nav_plane_AB(2)*pos(2)+nav_plane_AB(4))/(nav_plane_AB(2)*versore_son_NED(2)+versore_son_NED(1));
    t_BC = -(pos(1)+nav_plane_BC(2)*pos(2)+nav_plane_BC(4))/(nav_plane_BC(2)*versore_son_NED(2)+versore_son_NED(1));
    t_CD = -(pos(1)+nav_plane_CD(2)*pos(2)+nav_plane_CD(4))/(nav_plane_CD(2)*versore_son_NED(2)+versore_son_NED(1));
    t_DA = -(pos(1)+nav_plane_DA(2)*pos(2)+nav_plane_DA(4))/(nav_plane_DA(2)*versore_son_NED(2)+versore_son_NED(1));
    
    if t_AB < 0
        t_AB = inf;
    end
    if t_BC < 0
        t_BC = inf;
    end
    if t_CD < 0
        t_CD = inf;
    end
    if t_DA < 0
        t_DA = inf;
    end
           
    [dist, index] = min([t_AB t_BC t_CD t_DA]);
    dist = dist - 0.267;       %va tolto il raggio del robot rispetto al centro di massa
    
    switch index
        case 1
            plane = nav_plane_AB;
        case 2
            plane = nav_plane_BC;
        case 3
            plane = nav_plane_CD;
        case 4
            plane = nav_plane_DA;
        otherwise
            plane=[0 0 0 0];
            disp('errore nella intersezione del piano')
    end
    
end

function [H1, H2, H3]= calc_H_vect(pos, sonar, plane)

    H1 = sign(pos(1) + plane(4) + pos(2)*plane(2))/abs(sonar(1) + plane(2)*sonar(2));
    H2 = (plane(2)*sign(pos(1) + plane(4) + pos(2)*plane(2)))/abs(sonar(1) + plane(2)*sonar(2));   
    H3 = 0;
end

== matlab function sim_all/Navigation/Extended Kalman Filter/PREDIZIONE/Passo di Predizione ==
  data: x0 input; P0 input; x_k_1 input; u_k_1 input; x_k output; P_k_1 input; P_k output size=3 3; J input; L input; Q_k_1 input; nav_DT parameter; nav_flag_init input; nav_flag_init output
%% Passo di PREDIZIONE

function [x_k,  P_k, nav_flag_init] = prediction(x0, P0, x_k_1, u_k_1,  P_k_1, J, L, Q_k_1, nav_DT, nav_flag_init)
    
    x_k = zeros(3,1);
    P_k = zeros(3,3);

    % il valore di nav_flag_init all'inizio della simulazione é pari a 0
    % appena c'è il primo dato disponibile del GPS (insieme al profondimetro)
    % si assume quella come punto di inizializzazione del filtro.

    if nav_flag_init ~= 0      
        if nav_flag_init == 1
            x_k_1 = x0;
            P_k_1 = P0;
            nav_flag_init = 2;      % =2 così l'inizializzazione è fatta una sola volta.
        end
        
        %passo di predizione       
        x_k = x_k_1 + nav_DT*J*u_k_1;
        P_k = P_k_1 + L*Q_k_1*L';               %la matrice F è F = I
           
    end
end

== matlab function sim_all/Navigation/Extended Kalman Filter/Q_error/MATLAB Function4 ==
  data: Q input; Q_k_1 input; Q_k output; flag_AHRS input; flag_DVL input
%calcolo matrice Q
function Q_k = fcn(Q, Q_k_1, flag_AHRS, flag_DVL)

    Q_k = Q;
    
    K=10;
    if flag_DVL == 1
       Q_k = Q_k_1 + K*5*diag([0,0,0,(0.012)^2,(0.012)^2,(0.012)^2]);
    end
    
    if flag_AHRS == 1
       Q_k = Q_k_1 + K*50*diag([(0.0087)^2, (0.0087)^2, (0.0017)^2,0,0,0]);  
    end
        
end

== matlab function sim_all/Navigation/Gyro_check/MATLAB Function4 ==
  data: flag_gyro output; gyro_new input; gyro_now output; gyro_old input
% gestione di misura errata del giroscopio
function [flag_gyro, gyro_now] = fcn(gyro_new, gyro_old)

    if isnan(gyro_new(1,1)) || isnan(gyro_new(2,1)) || isnan(gyro_new(3,1))
        gyro_now = gyro_old;
        flag_gyro = 1;
        disp('Misura gyro non valida')
    else
        gyro_now = gyro_new;
        flag_gyro = 0;
    end  
end

== matlab function sim_all/Navigation/MATLAB Function ==
  data: u input; y output
function y = Wrap2pi(u)
y = [0;0;0];
coder.extrinsic('wrapToPi');
y = wrapToPi(u);
end

== matlab function sim_all/Navigation/NED2ECEF ==
  data: pos_es_NED input; pos_es_ECEF output; nav_lat0 parameter; nav_lon0 parameter; nav_h0 parameter
%%Blocco di conversione NED2ECEF

function pos_es_ECEF = pos_NED2ECEF(pos_es_NED,nav_lat0, nav_lon0, nav_h0)
     
    coder.extrinsic('evalin', 'wgs84Ellipsoid', 'ned2geodetic');
    pos_es_ECEF = zeros(3,1);
    depth = pos_es_NED(3); 
    
    [pos_es_ECEF(1),pos_es_ECEF(2),pos_es_ECEF(3)]= ned2geodetic(pos_es_NED(1),pos_es_NED(2),0,nav_lat0,nav_lon0,nav_h0,wgs84Ellipsoid);
    pos_es_ECEF(3) = depth;
end

== matlab function sim_all/Navigation/SOS_flag_generator/MATLAB Function ==
  data: P_es input; SOS output; DVL input; AHRS input; gyro input; contatore input size=3 1; contatore output
%% Generazione flag di emergenza
% 1. Assenza di segnali dai sensori per un determinato tempo

function [SOS, contatore] = SOS_flag(P_es, DVL, AHRS, gyro, contatore)
    SOS=0;
 
    soglia_P = 10; %[m^2]
    if P_es(1,1)+P_es(2,2) > soglia_P || P_es(3,3) > soglia_P
        SOS=1;
    end
    
    if DVL == 1 
        contatore(1) = contatore(1) + 1;
    else
        contatore(1) = 0;
    end
    
    if AHRS == 1 
        contatore(2) = contatore(2) + 1;
    else
        contatore(2) = 0;
    end
    
    if gyro == 1 
        contatore(3) = contatore(3) + 1;
    else
        contatore(3) = 0;
    end
    
    if max(contatore) > 50 %50 equivale a 5 secondi
        SOS=1;
    end
    
    

end

== matlab function sim_all/Mission_supervisor_v3/Mission_Supervisor/Immersione/MATLAB Function ==
  data: soglia_pos parameter; delta_current_immers output; delta_stato_immers output; Pos_d output size=3; Or_d output size=3; Pos_s input; depth parameter; punto_iniz_patt input; Or_in input; error_flag input; soglia_SOS_pos parameter; SOS parameter
function [delta_current_immers, delta_stato_immers, Pos_d, Or_d]=Immersione(soglia_pos, Pos_s, depth, punto_iniz_patt, Or_in, error_flag, soglia_SOS_pos, SOS)

    disp("Immersione");
    
    %% Unità di misura 
    
    % Pos_d, Pos_s, punto_iniz_patt, soglia_pos, soglia_SOS_pos            [deg, deg, m]
    % Or_d, Or_in                                                          [rad, rad, rad]
    % distanceFromWall, depth                                              [m]


    %% Inizializzazione variabili
    
    % Utilizzata durante la permanenza nello stato corrente
    delta_stato_immers = 0;
    
    pronti = false; 
    
    %% Preparazione dei riferimenti da fornire ai blocchi successivi
    
    % Posizione da raggiungere
    Pos_d = [punto_iniz_patt(1); punto_iniz_patt(2); depth];
                                                                            %*****TEST******%
                                                                            %Pos_d = [43; 11; 0];
    
    % Orientazione da mantenere
    Or_d = Or_in;
    
    % Transizione di stato effettiva
    delta_current_immers = 103 - 102;  
        
       
    %% Verifiche
    
    % Verifica della corretta posizione
    if (abs(Pos_s(1) - Pos_d(1)) > soglia_SOS_pos(1) || ...
        abs(Pos_s(2) - Pos_d(2)) > soglia_SOS_pos(2))
    
        SOS = 1;
        disp("EMERGENZA:"); 
        
        if (abs(Pos_s(1) - Pos_d(1)) > soglia_SOS_pos(1))
            disp("Rilevato errore sulla posizione X");
        end
        
        if (abs(Pos_s(2) - Pos_d(2)) > soglia_SOS_pos(2))
            disp("Rilevato errore sulla posizione Y");
        end

    end
    
    if error_flag == 1
        disp("EMERGENZA: errore segnalato dagli altri sottosistemi");
        SOS = 1;
    end
    
    % Si verifica di aver raggiunto la profondità desiderata 
    if (SOS == 0 && ...
        abs(Pos_s(3) - Pos_d(3)) < soglia_pos(3))
    
        pronti = true;
    end
    
    
    %% Decisione dello stato successivo
    
    if pronti == true
        
        delta_stato_immers = 104 - 103; % Transizione eseguita correttamente
    end 
    if SOS == 1
            
            delta_stato_immers = 301 - 103; % Transizione nello stato di emergenza
    end
    % Si rimane nello stato corrente

end
